simulink model "Mdl_Examle01_d"  (Simulink 6.1)
settings: Solver=ode4  StartTime=0.0  StopTime=10  FixedStep=0.01  RelTol=1e-3
values from neighbouring files (symbols this model uses):
  A = [-0.022872,0.34878,0;0,0,1;-0.458771,0.458771,0.025332]    [Example01.m]    (also in Example01_b.m = [ -0.022872   0.34878   0; Example01_c.m = [ -0.022872   0.34878   0; Example01_d.m = [ -0.022872   0.34878   0)
  B = [0.167254,0.167254;0,0;8.40879,8.40879]    [Example01.m]    (also in Example01_b.m = [ 0.167254   0.167254; Example01_c.m = [ 0.167254   0.167254; Example01_d.m = [ 0.167254   0.167254)
  C = eye(3)    [Example01.m]    (also in Example01_b.m = [0 1 0;0 0 1]; Example01_c.m = [0 1 0;0 0 1]; Example01_d.m)
  D_actuator = (A*w_actuator-lamda_actuator*w_actuator)*Cw_actuator_pinv+E*(I-Cfi_actuator*Cfi_actuator_pinv)    [Example01.m]    (also in Example01_b.m = ( A*w_actuator - lamda_actuator*w_actuator )*Cw_actuator_pin; Example01_c.m = K_couple'; Example01_d.m = K_couple')
  fi_actuator = [-0.167254;0;-8.40879]    [Example01.m]    (also in Example01_b.m = [ -0.167254; Example01_c.m = [ -0.167254; Example01_d.m = [ -0.167254)
libraries: simulink x1
settings Model: LastModifiedBy=Administrator
settings DebuggingCC: SolverPrmCheckMsg=warning

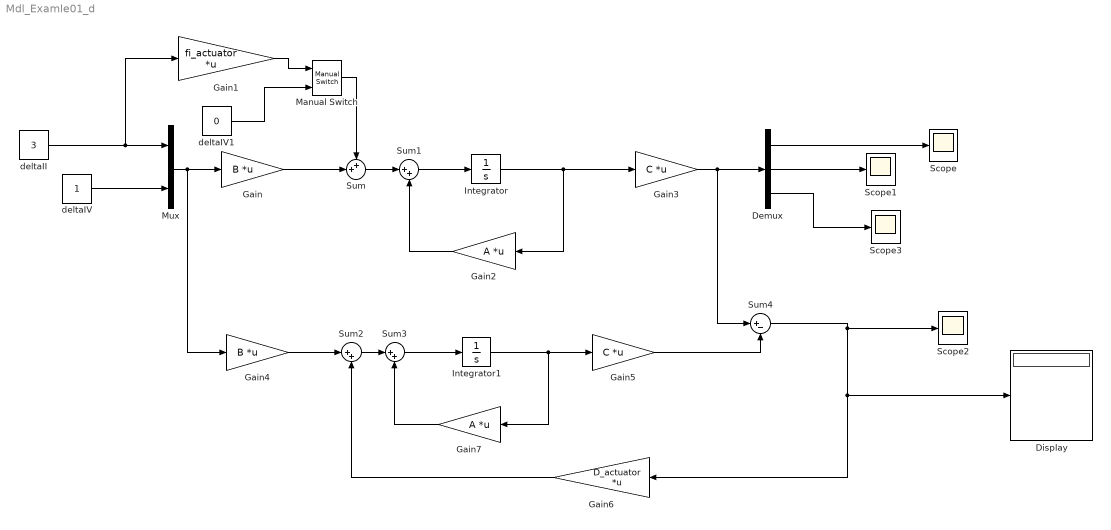
== system Mdl_Examle01_d ==
  Demux : Demux  Outputs=3
  Display : Display
  Gain : Gain  Gain=B  Multiplication=Matrix(K*u)
  Gain1 : Gain  Gain=fi_actuator  Multiplication=Matrix(K*u)
  Gain2 : Gain  Orientation=left  Gain=A  Multiplication=Matrix(K*u)
  Gain3 : Gain  Gain=C  Multiplication=Matrix(K*u)
  Gain4 : Gain  Gain=B  Multiplication=Matrix(K*u)
  Gain5 : Gain  Gain=C  Multiplication=Matrix(K*u)
  Gain6 : Gain  Orientation=left  Gain=D_actuator  Multiplication=Matrix(K*u)
  Gain7 : Gain  Orientation=left  Gain=A  Multiplication=Matrix(K*u)
  Integrator : Integrator  InitialCondition=[0;1;2]
  Integrator1 : Integrator
  Manual Switch : simulink/Signal Routing/Manual Switch  sw=1  action=0
  Mux : Mux  Inputs=2
  Scope{,1..3} (4 alike) : Scope
      Scope2 settings: SaveName=ScopeData2
      Scope3 settings: SaveName=ScopeData3
  Sum : Sum  Inputs=++|
  Sum1 : Sum  Inputs=|++
  Sum2 : Sum  Inputs=|++
  Sum3 : Sum  Inputs=|++
  Sum4 : Sum  Inputs=|+-
  deltaII : Constant  Value=3
  deltaIV : Constant
  deltaIV1 : Constant  Value=0
  wires:
  deltaII/1 -> Mux/1, Gain1/1
  deltaIV/1 -> Mux/2
  Mux/1 -> Gain/1, Gain4/1
  Gain/1 -> Sum/2
  Sum/1 -> Sum1/1
  Sum1/1 -> Integrator/1
  Integrator/1 -> Gain2/1, Gain3/1
  Gain2/1 -> Sum1/2
  Gain3/1 -> Demux/1, Sum4/1
  Demux/1 -> Scope/1
  Demux/2 -> Scope1/1
  Gain4/1 -> Sum2/1
  Sum2/1 -> Sum3/1
  Integrator1/1 -> Gain5/1, Gain7/1
  Sum3/1 -> Integrator1/1
  Gain5/1 -> Sum4/2
  Sum4/1 -> Scope2/1, Gain6/1, Display/1
  Gain6/1 -> Sum2/2
  Gain7/1 -> Sum3/2
  Demux/3 -> Scope3/1
  Gain1/1 -> Manual Switch/1
  Manual Switch/1 -> Sum/1
  deltaIV1/1 -> Manual Switch/2
